simulink model "test9"  (R2014b)
settings: Solver=ode45  StartTime=0.0  StopTime=.5  RelTol=1e-3
undefined symbols (not defined in the file or in its folder): i
libraries: dsparch4 x3, dspsigops x2
settings Model: Creator=Ben  LastModifiedBy=Ben

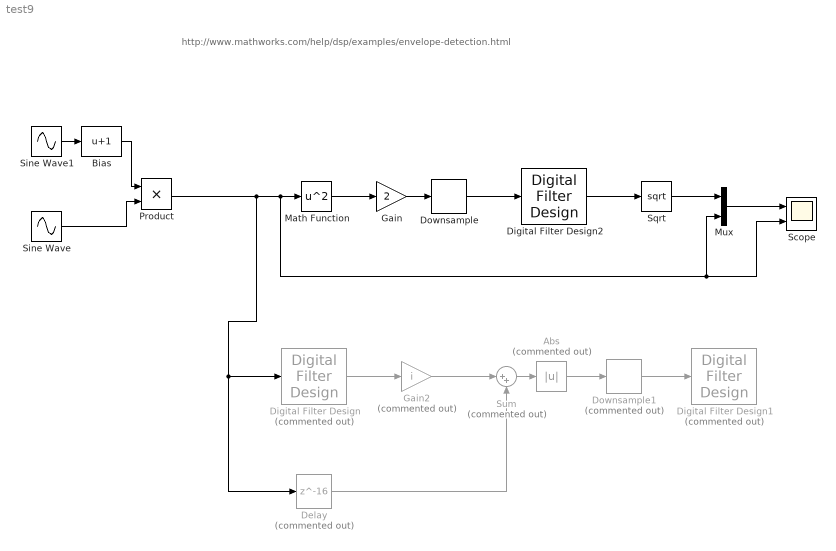
== system test9 ==
  note: http://www.mathworks.com/help/dsp/examples/envelope-detection.html
  Abs : Abs  Commented=on
  Bias : Bias  Bias=1
  Delay : Delay  Commented=on  DelayLength=16  InitialCondition=0
  Digital Filter Design : dsparch4/Digital Filter Design  Commented=on  mwdsp_browser_bugfix_var=off
  Digital Filter Design1 : dsparch4/Digital Filter Design  Commented=on  mwdsp_browser_bugfix_var=off
  Digital Filter Design2 : dsparch4/Digital Filter Design  mwdsp_browser_bugfix_var=off
  Downsample : dspsigops/Downsample  N=15  phase=0  RateOptions=Enforce single-rate processing  smode=Allow multirate  fmode=Maintain input frame size  ic=0
  Downsample1 : dspsigops/Downsample  Commented=on  N=15  phase=0  RateOptions=Enforce single-rate processing  smode=Allow multirate  fmode=Maintain input frame size  ic=0
  Gain : Gain  Gain=2
  Gain2 : Gain  Commented=on  Gain=i
  Math Function : Math  Operator=square  SaturateOnIntegerOverflow=on
  Mux : Mux  Inputs=2
  Product : Product
  Scope : Scope  NumInputPorts=2
      settings: YMin=-5~-5  YMax=5~5
  Sine Wave : Sin  Frequency=200*2*pi  SampleTime=1/22050
  Sine Wave1 : Sin  Amplitude=.4  Frequency=10*2*pi  SampleTime=1/22050
  Sqrt : Sqrt  SaturateOnIntegerOverflow=on
  Sum : Sum  Commented=on  Inputs=|++
  wires:
  Sine Wave1/1 -> Bias/1
  Sine Wave/1 -> Product/2
  Math Function/1 -> Gain/1
  Gain/1 -> Downsample/1
  Downsample/1 -> Digital Filter Design2/1
  Digital Filter Design/1 -> Gain2/1
  Delay/1 -> Sum/2
  Sum/1 -> Abs/1
  Abs/1 -> Downsample1/1
  Downsample1/1 -> Digital Filter Design1/1
  Gain2/1 -> Sum/1
  Product/1 -> Digital Filter Design/1, Delay/1, Math Function/1, Scope/2, Mux/2
  Bias/1 -> Product/1
  Mux/1 -> Scope/1
  Sqrt/1 -> Mux/1
  Digital Filter Design2/1 -> Sqrt/1
